simulink model "Verhulst"  (R2024b)
settings: Solver=VariableStepAuto  StartTime=0.0  StopTime=0.8  RelTol=1e-3
settings Model: Creator=max  LastModifiedBy=max

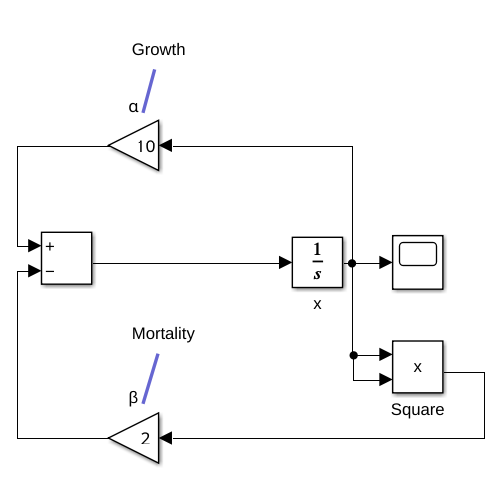
[thumbnail: Simulink's stored preview of the top-level diagram]
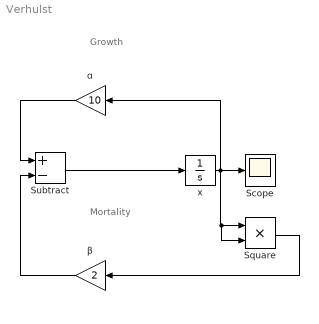
== system Verhulst ==
  note: Mortality
  note: Growth
  Scope : Scope
  Square : Product
  Subtract : Sum  Inputs=+-
  x : Integrator  InitialCondition=0.1
  ɑ : Gain  Gain=10
  β : Gain  Gain=2
  wires:
  x/1 -> Scope/1, ɑ/1, Square/2, Square/1
  Square/1 -> β/1
  ɑ/1 -> Subtract/1
  β/1 -> Subtract/2
  Subtract/1 -> x/1
